simulink model "simulation"  (R2019b)
settings: Solver=FixedStepDiscrete  StartTime=0.0  StopTime=25  FixedStep=Ts_proc  RelTol=1e-3
model workspace: external: MAT-File (data not in the file)
values from neighbouring files (symbols this model uses):
  CCR_init = CCR_max/2    [simulation_init.m]
  delay_input = 0    [simulation_init.m]
  dpole_cut = exp(-w_cut*Ts_ctrl)    [simulation_init.m]
  par_ctrl = Simulink.Parameter(par_ctrl)    [simulation_init.m]
  par_dn = Simulink.Parameter(par_dn)    [simulation_init.m]
  q_init = [0;pi]    [simulation_init.m]
  th_lim = 35/180*pi    (= 0.610865238198)    [simulation_init.m]
  Ts_ctrl = 5e-3    (= 0.005)    [simulation_init.m]
  Ts_proc = 1e-3    (= 0.001)    [simulation_init.m]
undefined symbols (not defined in the file or in its folder): bma, bp, CCR_max, DiscIntNeverNeededParam, encoder_res, eta_g, g, J0, Jp, Ke, Kg, Kt, Larm, Lm, lp, Lp, mp, Rm, volt_max
settings Model: OrderedModelArguments=off  Creator=Simone  LastModifiedBy=simone
settings OptimizationCC: DefaultParameterBehavior=Inlined  UseDivisionForNetSlopeComputation=on  GainParamInheritBuiltInType=on  UseFloatMulNetSlope=on  DefaultUnderspecifiedDataType=single  UseSpecifiedMinMax=on  InlineInvariantSignals=on  PassReuseOutputArgsAs=Individual arguments  ZeroExternalMemoryAtStartup=off  ZeroInternalMemoryAtStartup=off  NoFixptDivByZeroProtection=on  EfficientFloat2IntCast=on  LifeSpan=inf  OptimizeBlockOrder=speed  EfficientTunableParamExpr=on
settings DebuggingCC: SignalInfNanChecking=warning  ParameterTunabilityLossMsg=error  UniqueDataStoreMsg=error  AssertControl=DisableAll  SFUndirectedBroadcastEventsDiag=error
settings HardwareCC: ProdBitPerLong=64  ProdLongLongMode=on  ProdHWDeviceType=Intel->x86-64 (Linux 64)
settings SFSimCC: SimBuildMode=sf_nonincremental_build  CompileTimeRecursionLimit=0  EnableRuntimeRecursion=off  MATLABDynamicMemAlloc=off
settings RTWCC: SystemTargetFile=ert.tlc  GenCodeOnly=on  PackageGeneratedCodeAndArtifacts=on  TemplateMakefile=ert_default_tmf  GenerateReport=on  Toolchain=GNU gcc/g++ | gmake (64-bit Linux)  BuildConfiguration=Faster Runs  IncludeHyperlinkInReport=on  LaunchReport=on  GenerateTraceInfo=on  GenerateTraceReport=on  GenerateTraceReportSl=on  GenerateTraceReportSf=on  GenerateTraceReportEml=on  CheckMdlBeforeBuild=Error
settings CodeAppCC: ForceParamTrailComments=on  IgnoreCustomStorageClasses=off  IgnoreTestpoints=on  OperatorAnnotations=on  SimulinkDataObjDesc=on  SFDataObjDesc=on  MATLABFcnDesc=on  InsertBlockDesc=on  StateflowObjectComments=on  MATLABSourceComments=on  EnableCustomComments=on  ReqsInCode=on
settings ERTTargetCC: TargetLangStandard=C99 (ISO)  UtilityFuncGeneration=Shared location  CombineSignalStateStructs=on  SuppressErrorStatus=on  SupportNonFinite=off  ParenthesesLevel=Minimum  CastingMode=Standards  GenerateSharedConstants=off  InlinedParameterPlacement=NonHierarchical  ERTCustomFileTemplate=example_file_process.tlc  EnableSignedLeftShifts=off  EnableSignedRightShifts=off

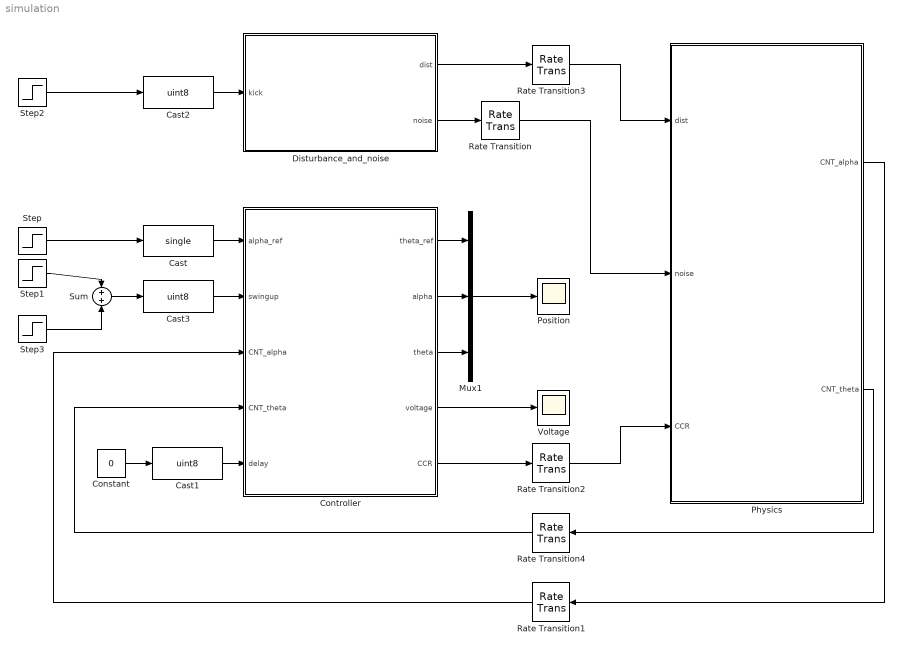
== system simulation ==
  Cast : DataTypeConversion  OutDataTypeStr=single
  Cast1 : DataTypeConversion  OutDataTypeStr=uint8
  Cast2 : DataTypeConversion  OutDataTypeStr=uint8
  Cast3 : DataTypeConversion  OutDataTypeStr=uint8
  Constant : Constant  Value=0
  Controller : Subsystem  TreatAsAtomicUnit=on  RTWFcnName=controller
      settings: RTWSystemCode=Nonreusable function  RTWFcnNameOpts=User specified  RTWFileNameOpts=Use function name  FunctionInterfaceSpec=Allow arguments
  Disturbance_and_noise : Subsystem  TreatAsAtomicUnit=on  RTWFcnName=disturbance_and_noise
      settings: RTWSystemCode=Nonreusable function  RTWFcnNameOpts=User specified  RTWFileNameOpts=Use function name  FunctionInterfaceSpec=Allow arguments
  Mux1 : Mux  Inputs=3
  Physics : Subsystem  TreatAsAtomicUnit=on  RTWFcnName=physics
      settings: RTWSystemCode=Nonreusable function  RTWFcnNameOpts=User specified  RTWFileNameOpts=Use function name  FunctionInterfaceSpec=Allow arguments
  Position : Scope
  Rate Transition : RateTransition  InitialCondition=single([0;0])  OutPortSampleTime=Ts_proc
  Rate Transition1 : RateTransition  InitialCondition=single(fix(q_init(1)/(2*pi)*encoder_res))  OutPortSampleTime=Ts_ctrl
  Rate Transition2 : RateTransition  InitialCondition=CCR_init  OutPortSampleTime=Ts_proc
  Rate Transition3 : RateTransition  InitialCondition=single(0)  OutPortSampleTime=Ts_proc
  Rate Transition4 : RateTransition  InitialCondition=single(fix(q_init(2)/(2*pi)*encoder_res))  OutPortSampleTime=Ts_ctrl
  Step : Step  Time=20  Before=180  After=0  SampleTime=Ts_ctrl
  Step1 : Step  Time=4  SampleTime=Ts_ctrl
  Step2 : Step  Time=16  SampleTime=Ts_ctrl
  Step3 : Step  Time=20  After=-1  SampleTime=Ts_ctrl
  Sum : Sum  Inputs=+|+
  Voltage : Scope
  wires:
  Physics/1(CNT_alpha) -> Rate Transition1/1
  Controller/5(CCR) -> Rate Transition2/1
  Disturbance_and_noise/2(noise) -> Rate Transition/1
  Step/1 -> Cast/1
  Disturbance_and_noise/1(dist) -> Rate Transition3/1
  Step1/1 -> Sum/1
  Step2/1 -> Cast2/1
  Step3/1 -> Sum/2
  Controller/1(theta_ref) -> Mux1/1
  Rate Transition2/1 -> Physics/3(CCR)
  Rate Transition3/1 -> Physics/1(dist)
  Rate Transition1/1 -> Controller/3(CNT_alpha)
  Mux1/1 -> Position/1
  Controller/2(alpha) -> Mux1/2
  Controller/3(theta) -> Mux1/3
  Constant/1 -> Cast1/1
  Rate Transition/1 -> Physics/2(noise)
  Physics/2(CNT_theta) -> Rate Transition4/1
  Rate Transition4/1 -> Controller/4(CNT_theta)
  Controller/4(voltage) -> Voltage/1
  Cast/1 -> Controller/1(alpha_ref)
  Cast1/1 -> Controller/5(delay)
  Cast2/1 -> Disturbance_and_noise/1(kick)
  Cast3/1 -> Controller/2(swingup)
  Sum/1 -> Cast3/1

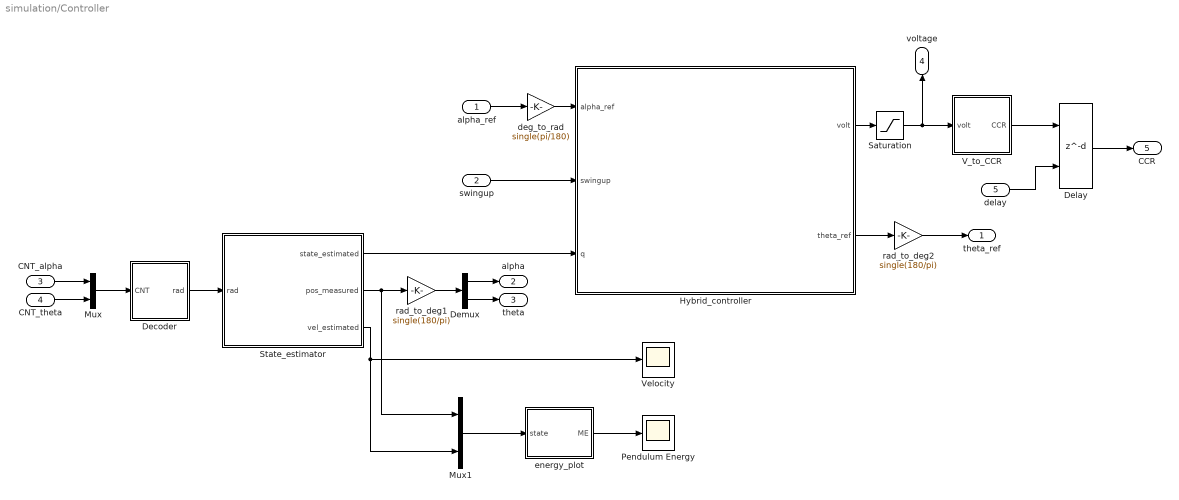
== system simulation/Controller ==
  alpha_ref : Inport
  swingup : Inport  Port=2
  CNT_alpha : Inport  Port=3
  CNT_theta : Inport  Port=4
  delay : Inport  Port=5
  Decoder : Subsystem
  Delay : Delay  DelayLengthSource=Input port  DelayLength=delay_input  DelayLengthUpperLimit=255  InitialCondition=CCR_init
      settings: InputPortMap=u0,p1
  Demux : Demux  Outputs=2
  Hybrid_controller : Stateflow chart  BlockKeywords=__PRM__SERIALIZED__DATA__:Stateflow Chart,Stateflow Diagram  TreatAsAtomicUnit=on
  Mux : Mux  Inputs=2
  Mux1 : Mux  Inputs=2
  Pendulum Energy : Scope
  Saturation : Saturate  UpperLimit=volt_max  LowerLimit=-volt_max
  State_estimator : Subsystem
  V_to_CCR : Subsystem
  Velocity : Scope
  deg_to_rad : Gain  Gain=single(pi/180)
  energy_plot : MATLAB Function
  rad_to_deg1 : Gain  Gain=single(180/pi)
  rad_to_deg2 : Gain  Gain=single(180/pi)
  theta_ref : Outport
  alpha : Outport  Port=2
  theta : Outport  Port=3
  voltage : Outport  Port=4
  CCR : Outport  Port=5
  wires:
  Hybrid_controller/1(volt) -> Saturation/1
  V_to_CCR/1(CCR) -> Delay/1
  State_estimator/2(pos_measured) -> Mux1/1, rad_to_deg1/1
  CNT_alpha/1 -> Mux/1
  Decoder/1(rad) -> State_estimator/1(rad)
  alpha_ref/1 -> deg_to_rad/1
  swingup/1 -> Hybrid_controller/2(swingup)
  Saturation/1 -> V_to_CCR/1(volt), voltage/1
  Delay/1 -> CCR/1
  Hybrid_controller/2(theta_ref) -> rad_to_deg2/1
  rad_to_deg1/1 -> Demux/1
  rad_to_deg2/1 -> theta_ref/1
  Demux/1 -> alpha/1
  Demux/2 -> theta/1
  Mux/1 -> Decoder/1(CNT)
  CNT_theta/1 -> Mux/2
  delay/1 -> Delay/2
  deg_to_rad/1 -> Hybrid_controller/1(alpha_ref)
  Mux1/1 -> energy_plot/1(state)
  energy_plot/1(ME) -> Pendulum Energy/1
  State_estimator/3(vel_estimated) -> Velocity/1, Mux1/2
  State_estimator/1(state_estimated) -> Hybrid_controller/3(q)

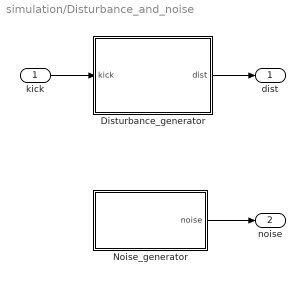
== system simulation/Disturbance_and_noise ==
  kick : Inport
  Disturbance_generator : Stateflow chart  BlockKeywords=__PRM__SERIALIZED__DATA__:Stateflow Chart,Stateflow Diagram  TreatAsAtomicUnit=on
  Noise_generator : Subsystem
  dist : Outport
  noise : Outport  Port=2
  wires:
  Noise_generator/1(noise) -> noise/1
  Disturbance_generator/1(dist) -> dist/1
  kick/1 -> Disturbance_generator/1(kick)

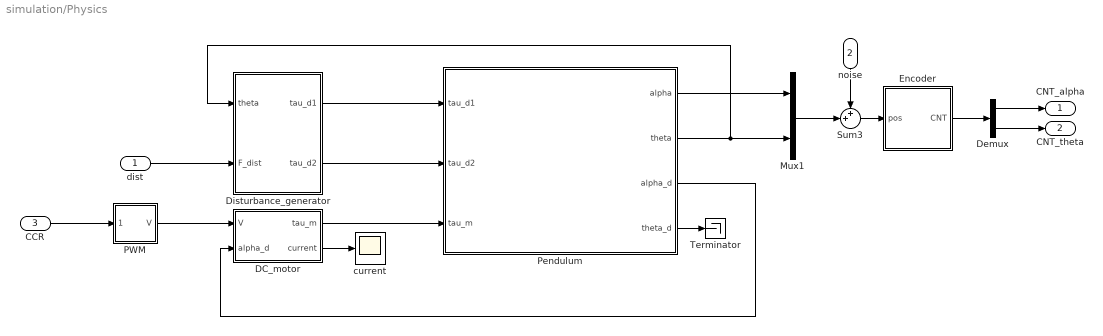
== system simulation/Physics ==
  dist : Inport
  noise : Inport  Port=2
  CCR : Inport  Port=3
  DC_motor : Subsystem
  Demux : Demux  Outputs=2
  Disturbance_generator : Subsystem
  Encoder : Subsystem
  Mux1 : Mux  Inputs=2
  PWM : Subsystem
  Pendulum : Subsystem
  Sum3 : Sum  Inputs=++|
  Terminator : Terminator
  current : Scope
  CNT_alpha : Outport
  CNT_theta : Outport  Port=2
  wires:
  PWM/1(V) -> DC_motor/1(V)
  Pendulum/3(alpha_d) -> DC_motor/2(alpha_d)
  DC_motor/2(current) -> current/1
  Pendulum/2(theta) -> Disturbance_generator/1(theta), Mux1/2
  Pendulum/1(alpha) -> Mux1/1
  Sum3/1 -> Encoder/1(pos)
  noise/1 -> Sum3/1
  Disturbance_generator/1(tau_d1) -> Pendulum/1(tau_d1)
  Disturbance_generator/2(tau_d2) -> Pendulum/2(tau_d2)
  DC_motor/1(tau_m) -> Pendulum/3(tau_m)
  CCR/1 -> PWM/1(CCR)
  dist/1 -> Disturbance_generator/2(F_dist)
  Mux1/1 -> Sum3/2
  Pendulum/4(theta_d) -> Terminator/1
  Encoder/1(CNT) -> Demux/1
  Demux/1 -> CNT_alpha/1
  Demux/2 -> CNT_theta/1

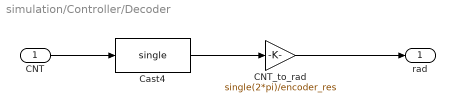
== system simulation/Controller/Decoder ==
  CNT : Inport
  CNT_to_rad : Gain  Gain=single(2*pi)/encoder_res
  Cast4 : DataTypeConversion  OutDataTypeStr=single
  rad : Outport
  wires:
  Cast4/1 -> CNT_to_rad/1
  CNT/1 -> Cast4/1
  CNT_to_rad/1 -> rad/1

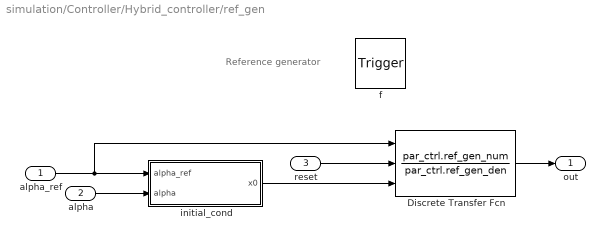
== system simulation/Controller/Hybrid_controller/ref_gen ==
  note: Reference generator
  alpha_ref : Inport  OutDataTypeStr=single  PortDimensions=1
  alpha : Inport  Port=2  OutDataTypeStr=single  PortDimensions=1
  reset : Inport  Port=3  OutDataTypeStr=int8  PortDimensions=1
  f : TriggerPort  TriggerType=function-call  VariantControl=(inherit)
      settings: CopyFcn=Stateflow.SLINSF.SimulinkMan.removeBlockPreDeleteFcn  PreDeleteFcn=Stateflow.SLINSF.SimulinkMan.unsafePredeleteFcn
  Discrete Transfer Fcn : DiscreteTransferFcn  Numerator=par_ctrl.ref_gen_num  Denominator=par_ctrl.ref_gen_den  InitialStatesSource=Input port  ExternalReset=Falling
      settings: InputPortMap=u0,r7,p5
  initial_cond : MATLAB Function
  out : Outport  OutDataTypeStr=single
  wires:
  alpha_ref/1 -> Discrete Transfer Fcn/1, initial_cond/1(alpha_ref)
  alpha/1 -> initial_cond/2(alpha)
  reset/1 -> Discrete Transfer Fcn/2
  Discrete Transfer Fcn/1 -> out/1
  initial_cond/1(x0) -> Discrete Transfer Fcn/3

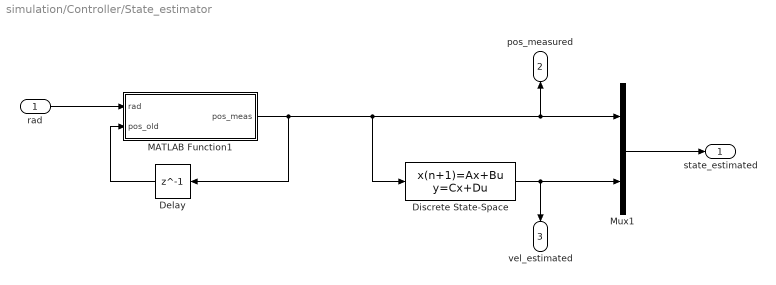
== system simulation/Controller/State_estimator ==
  rad : Inport
  Delay : Delay  DelayLength=1  InitialCondition=q_init
  Discrete State-Space : DiscreteStateSpace  A=dpole_cut*eye(2)  B=eye(2)  C=-1/single(Ts_ctrl)*(1-dpole_cut)^2*eye(2)  D=(1-dpole_cut)/single(Ts_ctrl)*eye(2)  InitialCondition=1/(1-dpole_cut)*eye(2)*q_init  SampleTime=Ts_ctrl
  MATLAB Function1 : MATLAB Function
  Mux1 : Mux  Inputs=2
  state_estimated : Outport
  pos_measured : Outport  Port=2
  vel_estimated : Outport  Port=3
  wires:
  Discrete State-Space/1 -> Mux1/2, vel_estimated/1
  Delay/1 -> MATLAB Function1/2(pos_old)
  rad/1 -> MATLAB Function1/1(rad)
  Mux1/1 -> state_estimated/1
  MATLAB Function1/1(pos_meas) -> Mux1/1, pos_measured/1, Discrete State-Space/1, Delay/1

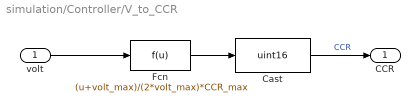
== system simulation/Controller/V_to_CCR ==
  volt : Inport
  Cast : DataTypeConversion  OutDataTypeStr=uint16  RndMeth=Round
  Fcn : Fcn  Expr=(u+volt_max)/(2*volt_max)*CCR_max
  CCR : Outport
  wires:
  Fcn/1 -> Cast/1
  Cast/1 -> CCR/1  "CCR"
  volt/1 -> Fcn/1

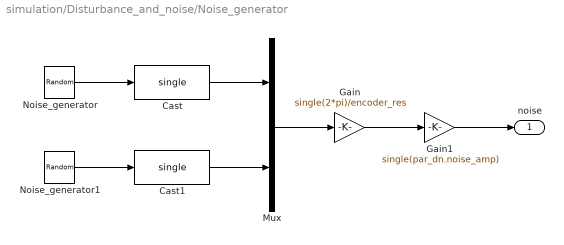
== system simulation/Disturbance_and_noise/Noise_generator ==
  Cast : DataTypeConversion  OutDataTypeStr=single
  Cast1 : DataTypeConversion  OutDataTypeStr=single
  Gain : Gain  Gain=single(2*pi)/encoder_res
  Gain1 : Gain  Gain=single(par_dn.noise_amp)
  Mux : Mux  Inputs=2
  Noise_generator : UniformRandomNumber  Seed=2342  SampleTime=Ts_ctrl
  Noise_generator1 : UniformRandomNumber  Seed=1558  SampleTime=Ts_ctrl
  noise : Outport
  wires:
  Mux/1 -> Gain/1
  Gain1/1 -> noise/1
  Gain/1 -> Gain1/1
  Noise_generator/1 -> Cast/1
  Noise_generator1/1 -> Cast1/1
  Cast/1 -> Mux/1
  Cast1/1 -> Mux/2

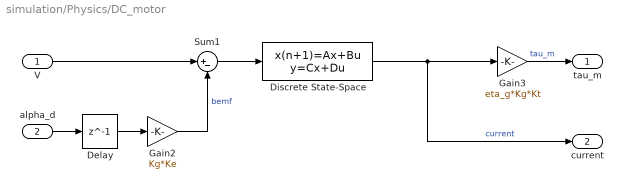
== system simulation/Physics/DC_motor ==
  V : Inport
  alpha_d : Inport  Port=2
  Delay : Delay  DelayLength=1  InitialCondition=0
  Discrete State-Space : DiscreteStateSpace  A=-(Rm*Ts_proc - 2*Lm)/(Rm*Ts_proc + 2*Lm)  B=Ts_proc/(2*Lm + Rm*Ts_proc)*(1-(Rm*Ts_proc - 2*Lm)/(Rm*Ts_proc + 2*Lm))  D=Ts_proc/(2*Lm + Rm*Ts_proc)  InitialCondition=single(0)  SampleTime=Ts_proc
  Gain2 : Gain  Gain=Kg*Ke
  Gain3 : Gain  Gain=eta_g*Kg*Kt
  Sum1 : Sum  Inputs=|+-
  tau_m : Outport
  current : Outport  Port=2
  wires:
  Delay/1 -> Gain2/1
  Gain3/1 -> tau_m/1  "tau_m"
  V/1 -> Sum1/1
  alpha_d/1 -> Delay/1
  Discrete State-Space/1 -> current/1, Gain3/1  "current"
  Sum1/1 -> Discrete State-Space/1
  Gain2/1 -> Sum1/2  "bemf"

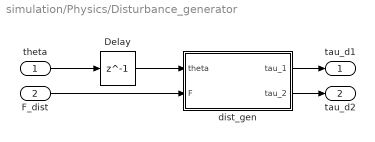
== system simulation/Physics/Disturbance_generator ==
  theta : Inport
  F_dist : Inport  Port=2
  Delay : Delay  DelayLength=1  InitialCondition=q_init(2)
  dist_gen : MATLAB Function
  tau_d1 : Outport
  tau_d2 : Outport  Port=2
  wires:
  dist_gen/1(tau_1) -> tau_d1/1
  dist_gen/2(tau_2) -> tau_d2/1
  F_dist/1 -> dist_gen/2(F)
  theta/1 -> Delay/1
  Delay/1 -> dist_gen/1(theta)

== system simulation/Physics/Encoder ==
  pos : Inport
  Cast2 : DataTypeConversion  OutDataTypeStr=uint16
  rad_to_CNT : MATLAB Function
  CNT : Outport
  wires:
  pos/1 -> rad_to_CNT/1(rad)
  Cast2/1 -> CNT/1
  rad_to_CNT/1(CNT) -> Cast2/1

== system simulation/Physics/PWM ==
  CCR : Inport
  Cast1 : DataTypeConversion  OutDataTypeStr=single
  Fcn1 : Fcn  Expr=volt_max*(2*u/CCR_max-1)
  V : Outport
  wires:
  CCR/1 -> Cast1/1
  Cast1/1 -> Fcn1/1
  Fcn1/1 -> V/1  "V"

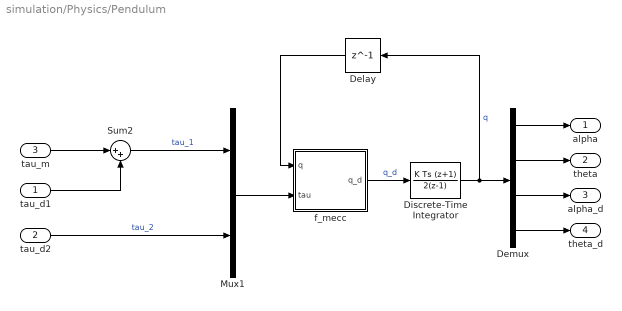
== system simulation/Physics/Pendulum ==
  tau_d1 : Inport
  tau_d2 : Inport  Port=2
  tau_m : Inport  Port=3
  Delay : Delay  DelayLength=1  InitialCondition=[q_init;0;0]
  Demux : Demux
  Discrete-Time Integrator : DiscreteIntegrator  IntegratorMethod=Integration: Trapezoidal  gainval=single(1.0)  InitialCondition=[q_init;0;0]  SampleTime=Ts_proc  ICPrevOutput=DiscIntNeverNeededParam  ICPrevScaledInput=DiscIntNeverNeededParam
  Mux1 : Mux  Inputs=2
  Sum2 : Sum  Inputs=|++
  f_mecc : MATLAB Function
  alpha : Outport
  theta : Outport  Port=2
  alpha_d : Outport  Port=3
  theta_d : Outport  Port=4
  wires:
  Delay/1 -> f_mecc/1(q)
  Demux/2 -> theta/1
  Demux/1 -> alpha/1
  Sum2/1 -> Mux1/1  "tau_1"
  tau_d2/1 -> Mux1/2  "tau_2"
  Discrete-Time Integrator/1 -> Delay/1, Demux/1  "q"
  Mux1/1 -> f_mecc/2(tau)
  f_mecc/1(q_d) -> Discrete-Time Integrator/1  "q_d"
  Demux/3 -> alpha_d/1
  Demux/4 -> theta_d/1
  tau_d1/1 -> Sum2/2
  tau_m/1 -> Sum2/1

== matlab function simulation/Physics/Encoder/rad_to_CNT ==
  data: rad input; CNT output; encoder_res parameter
function CNT = rad_to_CNT(rad,encoder_res)

CNT = floor(mod(rad,single(2*pi))/single(2*pi)*encoder_res);

== matlab function simulation/Physics/Pendulum/f_mecc ==
  data: q input single; q_d output single; tau input single; mp parameter; J0 parameter; Jp parameter; Larm parameter; lp parameter; g parameter; bma parameter; bp parameter
function q_d = f_mecc(q,tau,mp,J0,Jp,Larm,lp,g,bma,bp)
%#codegen

%    This function was generated by the Symbolic Math Toolbox version 8.4.
%    09-Dec-2019 19:45:31

al_d = q(3);
tau1 = tau(1);
tau2 = tau(2);
th = q(2);
th_d = q(4);
q_d = [al_d;th_d;((Jp.*tau1.*-2.0+Jp.*al_d.*bma.*2.0+Jp.^2.*al_d.*th_d.*sin(th.*2.0).*2.0+Larm.*lp.*mp.*tau2.*cos(th).*2.0-Larm.*bp.*lp.*mp.*th_d.*cos(th).*2.0+Larm.*g.*lp.^2.*mp.^2.*cos(th).*sin(th).*2.0-Jp.*Larm.*lp.*mp.*th_d.^2.*sin(th).*2.0+Jp.*Larm.*al_d.^2.*lp.*mp.*sin(th.*2.0).*cos(th)).*(-1.0./2.0))./(Jp.^2.*sin(th).^2+J0.*Jp-Larm.^2.*lp.^2.*mp.^2.*cos(th).^2);(J0.*tau2.*2.0+Jp.*tau2.*sin(th).^2.*2.0-J0.*bp.*th_d.*2.0+Jp.^2.*al_d.^2.*sin(th.*2.0).*sin(th).^2-Jp.*bp.*th_d.*sin(th).^2.*2.0+J0.*Jp.*al_d.^2.*sin(th.*2.0)+Jp.*g.*lp.*mp.*sin(th).^3.*2.0-Larm.*lp.*mp.*tau1.*cos(th).*2.0+J0.*g.*lp.*mp.*sin(th).*2.0+Larm.*al_d.*bma.*lp.*mp.*cos(th).*2.0-Larm.^2.*lp.^2.*mp.^2.*th_d.^2.*cos(th).*sin(th).*2.0+Jp.*Larm.*al_d.*lp.*mp.*th_d.*sin(th.*2.0).*cos(th).*2.0)./(Jp.^2.*sin(th).^2.*2.0+J0.*Jp.*2.0-Larm.^2.*lp.^2.*mp.^2.*cos(th).^2.*2.0)];

== matlab function simulation/Physics/Disturbance_generator/dist_gen ==
  data: theta input; F input; tau_1 output single; tau_2 output single; Larm parameter; Lp parameter
function [tau_1,tau_2] = dist_gen(theta,F,Larm,Lp)

tau_1 = F*Larm;
tau_2 = F*cos(theta)*Lp;

== matlab function simulation/Controller/State_estimator/MATLAB Function1 ==
  data: rad input single; pos_old input single; pos_meas output single
function pos_meas = pos_estim(rad,pos_old)

sect = @(th)mod(int8(floor(th/single(pi/2))),int8(4));

pos_meas = floor(pos_old/single(2*pi))*single(2*pi) +...
           mod(rad,single(2*pi));

for k=1:2
    if sect(pos_old(k)) == int8(3) && sect(rad(k)) == int8(0)
        pos_meas(k) = pos_meas(k) + single(2*pi);
    elseif sect(pos_old(k)) == int8(0) && sect(rad(k)) == int8(3)
        pos_meas(k) = pos_meas(k) - single(2*pi);
    end
end

== stateflow chart simulation/Controller/Hybrid_controller ==
  settings: updateMethod=DISCRETE  sampleTime=Ts_ctrl
  state PD_controller_up
    entry:
    ref_gen(alpha_ref,q(1),int8(1));
    theta_ref = round(q(2)/single(2*pi))*single(2*pi);
    entry, during:
    K = [par_ctrl.up_kp_alpha,...
    par_ctrl.up_kp_theta,...
    par_ctrl.up_kd_alpha,...
    par_ctrl.up_kd_theta];
    contr_pd;
  state Sliding_mode_controller
    during:
    theta_ref = round(q(2)/single(2*pi))*single(2*pi);
    state Idle
      during:
      volt = 0;
    state Swing_up
      entry, during:
      contr_su;
    Swing_up -> Idle : [energy(q) >= 0]
    (default) -> Idle
    Idle -> Swing_up : [energy(q) < 0]
  state PD_controller_down
    entry:
    ref_gen(alpha_ref,q(1),int8(1));
    entry, during:
    theta_ref = (round(q(2)/single(2*pi)+0.5)-0.5)*single(2*pi);
    K = [par_ctrl.down_kp_alpha,...
    single(0),...
    par_ctrl.down_kd_alpha,...
    single(0)];
    contr_pd;
  state out = ref_gen(alpha_ref,alpha,reset) [function]
  Sliding_mode_controller -> PD_controller_up [order 1] : [swingup == 1 &&...
      | abs(q(2)-round(q(2)/(2*pi))*2*pi) <= th_lim]
  PD_controller_up -> Sliding_mode_controller : [swingup == 0 ||...
      | abs(q(2)-round(q(2)/(2*pi))*2*pi) > th_lim]
  (default) -> Sliding_mode_controller
  PD_controller_down -> Sliding_mode_controller : [swingup == 1]
  Sliding_mode_controller -> PD_controller_down [order 2] : [swingup == 0]
  data: volt_max parameter; state function_input single; Jp parameter; Larm parameter; g parameter; lp parameter; mp parameter; ME function_output single; alpha_ref function_input single size=1; out function_output single; alpha function_input single size=1; reset function_input int8 size=1; alpha_ref input single; volt output single =single(0); swingup input uint8; q input single; th_lim parameter; K local single; par_ctrl parameter; theta_ref output single =single(pi)
  function contr_su:
    | % Swing-up controller
    | 
    | function contr_su
    | 
    | th = q(2);
    | th_d = q(4);
    | 
    | if th_d*cos(th) == 0
    |     sgn = sign(th);
    | else
    |     sgn = sign(th_d*cos(th));
    | end
    | 
    | volt = -volt_max*sgn;
  function contr_pd:
    | % PD controller with reference generator
    | 
    | function contr_pd
    | 
    | q_ref = [ref_gen(alpha_ref,q(1),int8(0)); theta_ref; 0; 0];
    | error = q_ref - q;
    | volt = K * error;
  function ME = energy(state):
    | % Mechanical energy calculation (kinetic + potential)
    | 
    | function ME = energy(state)
    | 
    | th = state(2);
    | al_d = state(3);
    | th_d = state(4);
    | 
    | ME = (Jp*al_d^2)/2 + (Jp*th_d^2)/2 + (Larm^2*al_d^2*mp)/2 - g*lp*mp - (Jp*al_d^2*cos(th)^2)/2 + g*lp*mp*cos(th) + Larm*al_d*lp*mp*th_d*cos(th);

== matlab function simulation/Controller/energy_plot ==
  data: state input; ME output; Jp parameter; Larm parameter; lp parameter; mp parameter; g parameter
function ME = energy(state,Jp,Larm,lp,mp,g)

th = state(2);
al_d = state(3);
th_d = state(4);

ME = (Jp*al_d^2)/2 + (Jp*th_d^2)/2 + (Larm^2*al_d^2*mp)/2 - g*lp*mp - (Jp*al_d^2*cos(th)^2)/2 + g*lp*mp*cos(th) + Larm*al_d*lp*mp*th_d*cos(th);

== stateflow chart simulation/Disturbance_and_noise/Disturbance_generator ==
  settings: updateMethod=DISCRETE  sampleTime=Ts_ctrl
  state Reset
    entry:
    dist = 0;
  state Off
  state On
    entry:
    dist = par_dn.dist_amp;
  (default) -> Reset
  On -> Reset : after(10,tick)
  Reset -> Off : [kick == 0]
  Off -> On : [kick == 1]
  data: kick input uint8; dist output single =single(0); par_dn parameter

== matlab function simulation/Controller/Hybrid_controller/ref_gen/initial_cond ==
  data: alpha_ref input; x0 output; alpha input; par_ctrl parameter
function x0 = initial_cond(alpha_ref, alpha, par_ctrl)

x0 = 1/par_ctrl.dpole_ref*(alpha/(1-par_ctrl.dpole_ref)-alpha_ref);
